simulink model "OffsetOutput_harness"  (Simulink 7.7)
settings: Solver=ode3  SolverMode=SingleTasking  StartTime=0.0  StopTime=25  FixedStep=.0005  RelTol=1e-3
PostLoadFcn:
  | cd '..';
  | PostLoadFcn;
  | cd 'harness';
InitFcn:
  | if signalbuilder('OffsetOutput_harness/Signal_Builder','activegroup') == 1
  |   CD_OFFSET_FUNCTION.DataType = 'uint8';
  |   CD_OFFSET_FUNCTION.Value = 255;
  | else
  |   CD_OFFSET_FUNCTION.DataType = 'uint8';
  |   CD_OFFSET_FUNCTION.Value = 0;
  | end
undefined symbols (not defined in the file): ACTIVE, BASE_ACTIVE, CD_PRECISION_REF_NOMINAL_VALUE, CD_VBATTERY_FILTER_DISPLAY_GAIN, CD_VBATTERY_FILTER_GAIN, CD_VBATTERY_GAIN, ENGINE_CRANKING, INIT_NORMAL, MXGTW_OFFSET, NON_FUNCTIONAL, ROD_ACTIVE, sigbuilder_block, srate, srate100, SYS_NORMAL
libraries: simulink x5, MX_Library x2
settings Model: Creator=smindema  LastModifiedBy=aliebel  CovPath=Offset  CovMetricSettings=dcmw  CovHTMLOptions=-aTS=1 -bRG=1 -bTC=1 -hTR=0 -nFC=0 -scm=1 -bcm=1 -xEv=0  covSaveCumulativeToWorkspaceVar=off  CovSaveSingleToWorkspaceVar=off
settings MATStruct: SampleTime=0.01  Offset=0  Priority=[1.0]
settings DataIOCC: LimitDataPoints=off  SaveOutput=off  SaveTime=off
settings OptimizationCC: BlockReduction=off  InlineParams=on  ExpressionFolding=off  StateBitsets=on  DataBitsets=on  UseTempVars=on  InitFltsAndDblsToZero=on  NoFixptDivByZeroProtection=on  EfficientFloat2IntCast=on  OptimizeModelRefInitCode=on
settings DebuggingCC: SaveWithParameterizedLinksMsg=none  MultiTaskDSMMsg=warning  MultiTaskCondExecSysMsg=none  IntegerOverflowMsg=none  ModelReferenceCSMismatchMessage=warning
settings HardwareCC: ProdBitPerInt=16  ProdBitPerPointer=16  ProdIntDivRoundTo=Floor  ProdEndianess=BigEndian  ProdWordSize=16  ProdHWDeviceType=Motorola HC12
settings ModelReferenceCC: ModelReferenceNumInstancesAllowed=Single
settings RTWCC: SystemTargetFile=ert.tlc  GenCodeOnly=on  TemplateMakefile=ert_default_tmf  Description=Real-Time Workshop Embedded Coder (no auto configuration)  GenerateReport=on  RetainRTWFile=on  ProcessScript=ert_make_rtw_hook  IncludeHyperlinkInReport=on  LaunchReport=on  IncludeERTFirstTime=on
settings RTWCC: CustomHeaderCode=|
  | #include "cpp_req_defines.h"
  | #include "hw_fin.h"
  | #include "cdata.h"
settings CodeAppCC: IgnoreCustomStorageClasses=off  DefineNamingRule=UpperCase
settings ERTTargetCC: TargetFcnLib=ansi_tfl_tmw.mat  FunctionExecutionProfile=off  MultiwordLength=2048  GenerateSampleERTMain=on  IncludeMdlTerminateFcn=off  SupportAbsoluteTime=off  SupportNonFinite=off  SupportComplex=off  PurelyIntegerCode=on  ERTCustomFileTemplate=gen_rtw_req_defines_h.tlc  GlobalDataDefinition=InSeparateSourceFile  GlobalDataReference=InSeparateHeaderFile  ConvertIfToSwitch=off

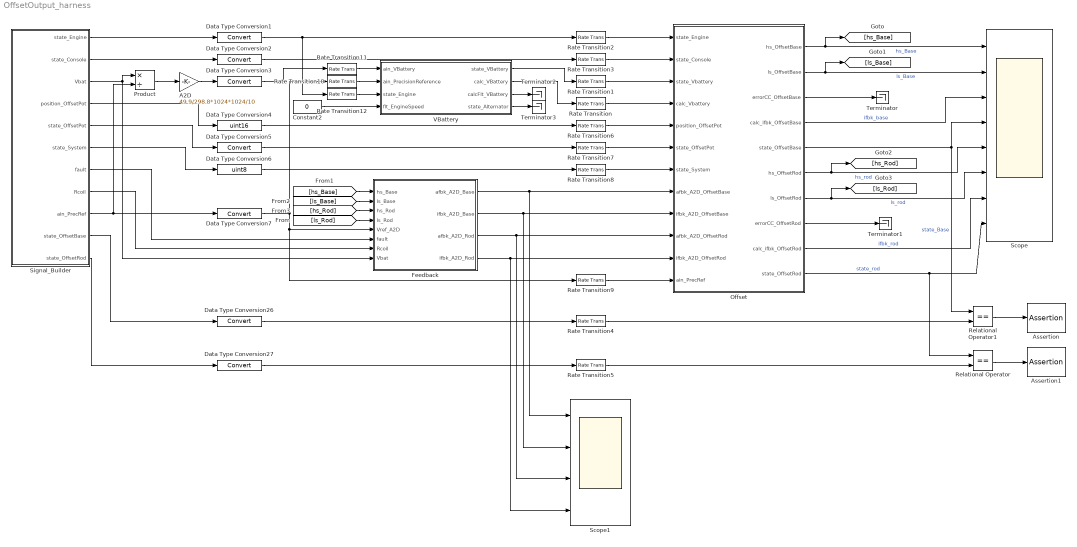
== system OffsetOutput_harness ==
  A2D : Gain  Gain=49.9/298.8*1024*1024/10  OutDataTypeStr=uint16
  Assertion : Assertion  Enabled=off
  Assertion1 : Assertion  Enabled=off
  Constant2 : Constant  Value=0  OutDataTypeStr=uint16
  Data Type Conversion{1..3,5,7,26..27} (7 alike) : DataTypeConversion
  Data Type Conversion4 : DataTypeConversion  OutDataTypeStr=uint16
  Data Type Conversion6 : DataTypeConversion  OutDataTypeStr=uint8
  Feedback : Subsystem
  Offset : Subsystem  TreatAsAtomicUnit=on  SystemSampleTime=srate  RTWFileName=mod_Outputs
      settings: RTWSystemCode=Function  RTWFcnNameOpts=Use subsystem name  RTWFileNameOpts=User specified
  Product : Product  Inputs=*/  RndMeth=Zero
  Rate Transition : RateTransition  X0=12
  Rate Transition1 : RateTransition  X0=8
  Rate Transition{2..12} (11 alike) : RateTransition
  Relational Operator : RelationalOperator  Operator===  OutDataTypeStr=boolean
  Relational Operator1 : RelationalOperator  Operator===  OutDataTypeStr=boolean
  Scope : Scope  NumInputPorts=8
      settings: TimeRange=50  YMin=0~0~0~0~0~0~0~0  YMax=0.3~1~1.25~1~0.4~1~1.5~1  DataFormat=Array
  Scope1 : Scope  NumInputPorts=4
      settings: TimeRange=100  YMin=0~0~0~0  YMax=6~10~6~60  SaveName=ScopeData2  DataFormat=Array
  Signal_Builder : Subsystem  Tag=STV Subsys  LoadFcn=sigbuilder_block('load');  StartFcn=sigbuilder_block('start');  StopFcn=sigbuilder_block('stop');  ClipboardFcn=sigbuilder_block('clipboard');  mask(Sigbuilder block){}
      mask help: Sigbuilder GUI
      mask init:
      | if ~strcmp(get_param(bdroot(gcbh),'SimulationStatus'),'stopped') tuvar = sigbuilder_block('maskInit'); end
      settings: CopyFcn=sigbuilder_block('copy');  DeleteFcn=sigbuilder_block('delete');  ModelCloseFcn=sigbuilder_block('modelClose');  PreSaveFcn=sigbuilder_block('preSave');  NameChangeFcn=sigbuilder_block('namechange');  OpenFcn=sigbuilder_block('open',[498.75 33 780.75 697.5 ]);  CloseFcn=sigbuilder_block('close');
      mask Display: plot(0,0,100,100,[10,10,40,40,10],[80,20,20,80,80],[40,10],[50,50], [40,27,10],[65,72,56],[40,25,25,10],[28,28,43,43]);
  Terminator{,1..3} (4 alike) : Terminator
  VBattery : Subsystem  TreatAsAtomicUnit=on  SystemSampleTime=srate100  RTWFileName=mod_Inputs
      settings: RTWSystemCode=Function  RTWFcnNameOpts=Use subsystem name  RTWFileNameOpts=User specified
  wires:
  Signal_Builder/2(state_Console) -> Data Type Conversion2/1
  Relational Operator/1 -> Assertion1/1
  Signal_Builder/1(state_Engine) -> Data Type Conversion1/1
  Signal_Builder/4(position_OffsetPot) -> Data Type Conversion4/1
  Relational Operator1/1 -> Assertion/1
  Signal_Builder/11(state_OffsetRod) -> Data Type Conversion27/1
  Data Type Conversion26/1 -> Rate Transition4/1
  Data Type Conversion27/1 -> Rate Transition5/1
  Data Type Conversion1/1 -> Rate Transition2/1, Rate Transition12/1
  Data Type Conversion2/1 -> Rate Transition3/1
  Signal_Builder/10(state_OffsetBase) -> Data Type Conversion26/1
  Data Type Conversion4/1 -> Rate Transition6/1
  Data Type Conversion5/1 -> Rate Transition7/1
  Data Type Conversion6/1 -> Rate Transition8/1
  Data Type Conversion7/1 -> Rate Transition10/1, Rate Transition9/1, Feedback/5(Vref_A2D)
  Signal_Builder/5(state_OffsetPot) -> Data Type Conversion5/1
  Signal_Builder/6(state_System) -> Data Type Conversion6/1
  Signal_Builder/9(ain_PrecRef) -> Data Type Conversion7/1, Product/2
  Offset/1(hs_OffsetBase) -> Scope/1, [hs_Base]  "hs_Base"
  Offset/2(ls_OffsetBase) -> Scope/2, [ls_Base]  "ls_Base"
  Offset/4(calc_ifbk_OffsetBase) -> Scope/3  "ifbk_base"
  Offset/5(state_OffsetBase) -> Scope/4, Relational Operator1/1  "state_Base"
  Offset/6(hs_OffsetRod) -> Scope/5, [hs_Rod]  "hs_rod"
  Offset/7(ls_OffsetRod) -> Scope/6, [ls_Rod]  "ls_rod"
  Offset/9(calc_ifbk_OffsetRod) -> Scope/7  "ifbk_rod"
  Offset/10(state_OffsetRod) -> Scope/8, Relational Operator/1  "state_rod"
  Offset/3(errorCC_OffsetBase) -> Terminator/1
  Offset/8(errorCC_OffsetRod) -> Terminator1/1
  VBattery/1(state_VBattery) -> Rate Transition1/1
  VBattery/2(calc_VBattery) -> Rate Transition/1
  VBattery/3(calcFlt_VBattery) -> Terminator2/1
  VBattery/4(state_Alternator) -> Terminator3/1
  Constant2/1 -> VBattery/4(flt_EngineSpeed)
  Signal_Builder/3(Vbat) -> Feedback/8(Vbat), Product/1
  A2D/1 -> Data Type Conversion3/1
  Data Type Conversion3/1 -> Rate Transition11/1
  Signal_Builder/7(fault) -> Feedback/6(fault)
  Signal_Builder/8(Rcoil) -> Feedback/7(Rcoil)
  [hs_Base] -> Feedback/1(hs_Base)
  [ls_Base] -> Feedback/2(ls_Base)
  [hs_Rod] -> Feedback/3(hs_Rod)
  [ls_Rod] -> Feedback/4(ls_Rod)
  Rate Transition1/1 -> Offset/3(state_Vbattery)
  Rate Transition/1 -> Offset/4(calc_Vbattery)
  Rate Transition2/1 -> Offset/1(state_Engine)
  Rate Transition3/1 -> Offset/2(state_Console)
  Rate Transition4/1 -> Relational Operator1/2
  Rate Transition5/1 -> Relational Operator/2
  Rate Transition6/1 -> Offset/5(position_OffsetPot)
  Rate Transition7/1 -> Offset/6(state_OffsetPot)
  Rate Transition8/1 -> Offset/7(state_System)
  Rate Transition9/1 -> Offset/12(ain_PrecRef)
  Rate Transition10/1 -> VBattery/2(ain_PrecisionReference)
  Rate Transition11/1 -> VBattery/1(ain_VBattery)
  Rate Transition12/1 -> VBattery/3(state_Engine)
  Feedback/1(afbk_A2D_Base) -> Offset/8(afbk_A2D_OffsetBase), Scope1/1
  Feedback/2(ifbk_A2D_Base) -> Offset/9(ifbk_A2D_OffsetBase), Scope1/2
  Feedback/3(afbk_A2D_Rod) -> Offset/10(afbk_A2D_OffsetRod), Scope1/3
  Feedback/4(ifbk_A2D_Rod) -> Offset/11(ifbk_A2D_OffsetRod), Scope1/4
  Product/1 -> A2D/1

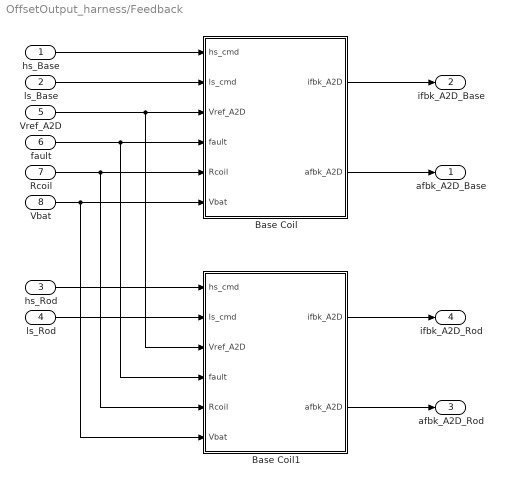
== system OffsetOutput_harness/Feedback ==
  hs_Base : Inport
  ls_Base : Inport  Port=2
  hs_Rod : Inport  Port=3
  ls_Rod : Inport  Port=4
  Vref_A2D : Inport  Port=5
  fault : Inport  Port=6
  Rcoil : Inport  Port=7
  Vbat : Inport  Port=8
  Base Coil : Subsystem
  Base Coil1 : Subsystem
  afbk_A2D_Base : Outport
  ifbk_A2D_Base : Outport  Port=2
  afbk_A2D_Rod : Outport  Port=3
  ifbk_A2D_Rod : Outport  Port=4
  wires:
  Base Coil/1(ifbk_A2D) -> ifbk_A2D_Base/1
  Base Coil/2(afbk_A2D) -> afbk_A2D_Base/1
  hs_Base/1 -> Base Coil/1(hs_cmd)
  ls_Base/1 -> Base Coil/2(ls_cmd)
  fault/1 -> Base Coil/4(fault), Base Coil1/4(fault)
  Rcoil/1 -> Base Coil/5(Rcoil), Base Coil1/5(Rcoil)
  Vbat/1 -> Base Coil/6(Vbat), Base Coil1/6(Vbat)
  Base Coil1/1(ifbk_A2D) -> ifbk_A2D_Rod/1
  Base Coil1/2(afbk_A2D) -> afbk_A2D_Rod/1
  hs_Rod/1 -> Base Coil1/1(hs_cmd)
  ls_Rod/1 -> Base Coil1/2(ls_cmd)
  Vref_A2D/1 -> Base Coil/3(Vref_A2D), Base Coil1/3(Vref_A2D)

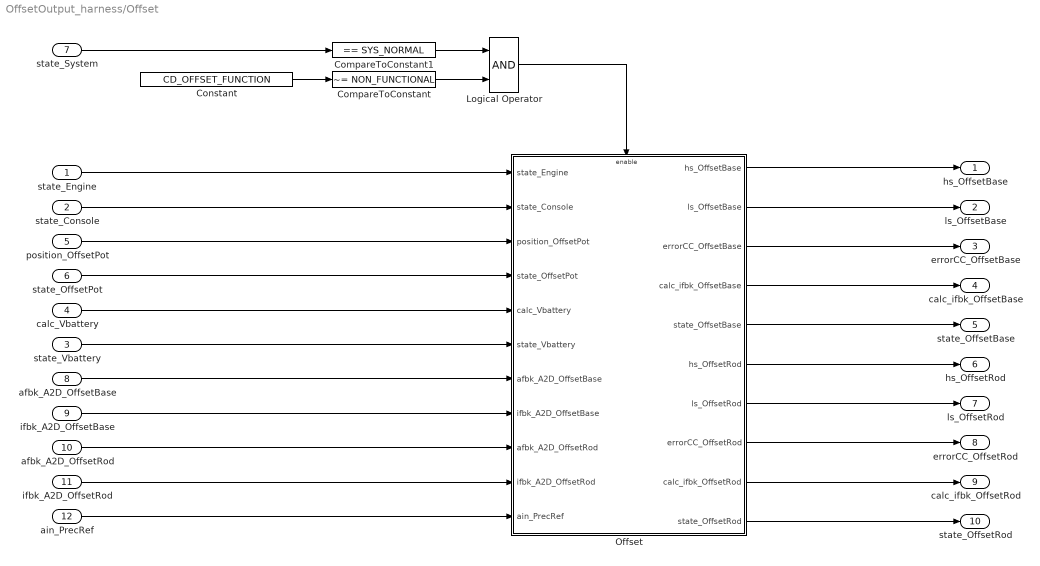
== system OffsetOutput_harness/Offset ==
  state_Engine : Inport
  state_Console : Inport  Port=2
  state_Vbattery : Inport  Port=3
  calc_Vbattery : Inport  Port=4
  position_OffsetPot : Inport  Port=5
  state_OffsetPot : Inport  Port=6
  state_System : Inport  Port=7
  afbk_A2D_OffsetBase : Inport  Port=8
  ifbk_A2D_OffsetBase : Inport  Port=9
  afbk_A2D_OffsetRod : Inport  Port=10
  ifbk_A2D_OffsetRod : Inport  Port=11
  ain_PrecRef : Inport  Port=12
  CompareToConstant : simulink/Logic and Bit Operations/Compare To Constant  SystemSampleTime=-1  relop=~=  const=NON_FUNCTIONAL  LogicOutDataTypeMode=boolean  ZeroCross=off
  CompareToConstant1 : simulink/Logic and Bit Operations/Compare To Constant  SystemSampleTime=-1  relop===  const=SYS_NORMAL  LogicOutDataTypeMode=boolean  ZeroCross=off
  Constant : Constant  Value=CD_OFFSET_FUNCTION
  Logical Operator : Logic  AllPortsSameDT=off  OutDataTypeStr=boolean
  Offset : Subsystem
  hs_OffsetBase : Outport  OutputWhenDisabled=reset  InitialOutput=[0]
  ls_OffsetBase : Outport  Port=2  OutputWhenDisabled=reset  InitialOutput=[0]
  errorCC_OffsetBase : Outport  Port=3  OutputWhenDisabled=reset  InitialOutput=[0]
  calc_ifbk_OffsetBase : Outport  Port=4  OutputWhenDisabled=reset  InitialOutput=[0]
  state_OffsetBase : Outport  Port=5  OutputWhenDisabled=reset  InitialOutput=[0]
  hs_OffsetRod : Outport  Port=6  OutputWhenDisabled=reset  InitialOutput=[0]
  ls_OffsetRod : Outport  Port=7  OutputWhenDisabled=reset  InitialOutput=[INIT_NORMAL]
  errorCC_OffsetRod : Outport  Port=8  OutputWhenDisabled=reset  InitialOutput=[0]
  calc_ifbk_OffsetRod : Outport  Port=9  OutputWhenDisabled=reset  InitialOutput=[INIT_NORMAL]
  state_OffsetRod : Outport  Port=10
  wires:
  state_System/1 -> CompareToConstant1/1
  CompareToConstant1/1 -> Logical Operator/1
  Constant/1 -> CompareToConstant/1
  CompareToConstant/1 -> Logical Operator/2
  Logical Operator/1 -> Offset/Enable
  state_Engine/1 -> Offset/1(state_Engine)
  state_Console/1 -> Offset/2(state_Console)
  position_OffsetPot/1 -> Offset/3(position_OffsetPot)
  state_OffsetPot/1 -> Offset/4(state_OffsetPot)
  calc_Vbattery/1 -> Offset/5(calc_Vbattery)
  state_Vbattery/1 -> Offset/6(state_Vbattery)
  afbk_A2D_OffsetBase/1 -> Offset/7(afbk_A2D_OffsetBase)
  ifbk_A2D_OffsetBase/1 -> Offset/8(ifbk_A2D_OffsetBase)
  afbk_A2D_OffsetRod/1 -> Offset/9(afbk_A2D_OffsetRod)
  ifbk_A2D_OffsetRod/1 -> Offset/10(ifbk_A2D_OffsetRod)
  Offset/1(hs_OffsetBase) -> hs_OffsetBase/1
  Offset/2(ls_OffsetBase) -> ls_OffsetBase/1
  Offset/3(errorCC_OffsetBase) -> errorCC_OffsetBase/1
  Offset/4(calc_ifbk_OffsetBase) -> calc_ifbk_OffsetBase/1
  Offset/5(state_OffsetBase) -> state_OffsetBase/1
  Offset/6(hs_OffsetRod) -> hs_OffsetRod/1
  Offset/7(ls_OffsetRod) -> ls_OffsetRod/1
  Offset/8(errorCC_OffsetRod) -> errorCC_OffsetRod/1
  Offset/9(calc_ifbk_OffsetRod) -> calc_ifbk_OffsetRod/1
  Offset/10(state_OffsetRod) -> state_OffsetRod/1
  ain_PrecRef/1 -> Offset/11(ain_PrecRef)

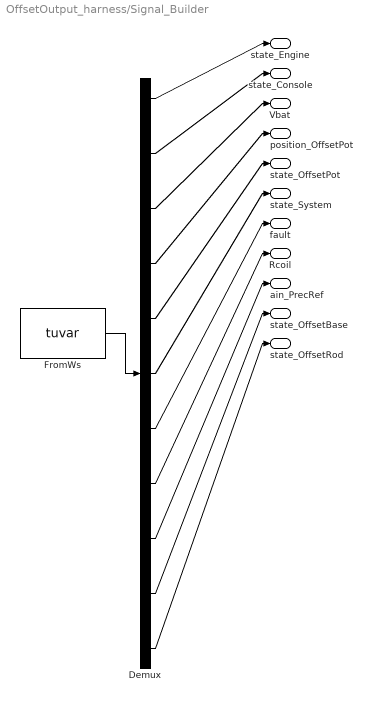
== system OffsetOutput_harness/Signal_Builder ==
  Demux : Demux  Tag=STV Demux  Outputs=11
  FromWs : FromWorkspace  Tag=STV FromWs  VariableName=tuvar  SampleTime=0  SigBuilderData=DataTag0  VnvData=DataTag1
      SigBuilderData=|
      | common.afterFinalStr = 'Extrapolate'
      | common.sampleTime = 0
      | dataSet(1).timeRange = [0 100]
      | dataSet(1).name = 'NonFunctional'
      | dataSet(2).timeRange = [0 100]
      | dataSet(2).name = 'Functional'
      | dataSet(3).timeRange = [0 100]
      | dataSet(3).name = 'Functional1'
      | dataSet(4).timeRange = [0 100]
      | dataSet(4).name = 'Open'
      | dataSet(5).timeRange = [0 100]
      | dataSet(5).name = 'STB'
      | dataSet(6).timeRange = [0 100]
      | dataSet(6).name = 'STG'
      | sbobj.Groups(1).Name = 'NonFunctional'
      | sbobj.Groups(1).Signals(1).Name = 'state_Engine'
      | sbobj.Groups(1).Signals(1).XData = [0 26 26 27 27 53 53 54 54 77 77 78 78 100]
      | sbobj.Groups(1).Signals(1).YData = [0 0 2 2 0 0 2 2 0 0 2 2 0 0]
      | sbobj.Groups(1).Signals(2).Name = 'state_Console'
      | sbobj.Groups(1).Signals(2).XData = [0 1 1 52 52 79 79 100]
      | sbobj.Groups(1).Signals(2).YData = [0 0 1 1 0 0 1 1]
      | sbobj.Groups(1).Signals(3).Name = 'Vbat'
      | sbobj.Groups(1).Signals(3).XData = [0 100]
      | sbobj.Groups(1).Signals(3).YData = [12 12]
      | sbobj.Groups(1).Signals(4).Name = 'position_OffsetPot'
      | sbobj.Groups(1).Signals(4).XData = [0 5 15 25 30 40 50 56 65 75 80 90 99 100]
      | sbobj.Groups(1).Signals(4).YData = [500 500 700 500 500 300 500 500 700 500 500 300 500 500]
      | sbobj.Groups(1).Signals(5).Name = 'state_OffsetPot'
      | sbobj.Groups(1).Signals(5).XData = [0 5 5 26 26 30 30 51 51 55 55 76 76 80 80 100]
      | sbobj.Groups(1).Signals(5).YData = [8 8 253 253 8 8 254 254 8 8 253 253 8 8 254 254]
      | sbobj.Groups(1).Signals(6).Name = 'state_System'
      | sbobj.Groups(1).Signals(6).XData = [0 78 78 100]
      | sbobj.Groups(1).Signals(6).YData = [1 1 2 2]
      | sbobj.Groups(1).Signals(7).Name = 'fault'
      | sbobj.Groups(1).Signals(7).XData = [0 100]
      | sbobj.Groups(1).Signals(7).YData = [0 0]
      | sbobj.Groups(1).Signals(8).Name = 'Rcoil'
      | sbobj.Groups(1).Signals(8).XData = [0 100]
      | sbobj.Groups(1).Signals(8).YData = [6 6]
      | sbobj.Groups(1).Signals(9).Name = 'ain_PrecRef'
      | sbobj.Groups(1).Signals(9).XData = [0 100]
      | sbobj.Groups(1).Signals(9).YData = [512 512]
      | sbobj.Groups(1).Signals(10).Name = 'state_OffsetBase'
      | sbobj.Groups(1).Signals(10).XData = [0 100]
      | sbobj.Groups(1).Signals(10).YData = [0 0]
      | sbobj.Groups(1).Signals(11).Name = 'state_OffsetRod'
      | sbobj.Groups(1).Signals(11).XData = [0 100]
      | sbobj.Groups(1).Signals(11).YData = [0 0]
      | sbobj.Groups(1).TimeRange = [0 100]
      | sbobj.Groups(2).Name = 'Functional'
      | sbobj.Groups(2).Signals(1).Name = 'state_Engine'
      | sbobj.Groups(2).Signals(1).XData = [0 26 26 27 27 53 53 54 54 77 77 78 78 100]
      | sbobj.Groups(2).Signals(1).YData = [0 0 2 2 0 0 2 2 0 0 2 2 0 0]
      | sbobj.Groups(2).Signals(2).Name = 'state_Console'
      | sbobj.Groups(2).Signals(2).XData = [0 1 1 52 52 79 79 100]
      | sbobj.Groups(2).Signals(2).YData = [0 0 1 1 0 0 1 1]
      | sbobj.Groups(2).Signals(3).Name = 'Vbat'
      | sbobj.Groups(2).Signals(3).XData = [0 100]
      | sbobj.Groups(2).Signals(3).YData = [12 12]
      | sbobj.Groups(2).Signals(4).Name = 'position_OffsetPot'
      | sbobj.Groups(2).Signals(4).XData = [0 5 15 25 30 40 50 56 65 75 80 90 99 100]
      | sbobj.Groups(2).Signals(4).YData = [500 500 700 500 500 300 500 500 700 500 500 300 500 500]
      | sbobj.Groups(2).Signals(5).Name = 'state_OffsetPot'
      | sbobj.Groups(2).Signals(5).XData = [0 5 5 26 26 30 30 51 51 55 55 76 76 80 80 100]
      | sbobj.Groups(2).Signals(5).YData = [8 8 253 253 8 8 254 254 8 8 253 253 8 8 254 254]
      | sbobj.Groups(2).Signals(6).Name = 'state_System'
      | sbobj.Groups(2).Signals(6).XData = [0 78 78 100]
      | sbobj.Groups(2).Signals(6).YData = [1 1 2 2]
      | sbobj.Groups(2).Signals(7).Name = 'fault'
      | sbobj.Groups(2).Signals(7).XData = [0 100]
      | sbobj.Groups(2).Signals(7).YData = [0 0]
      | sbobj.Groups(2).Signals(8).Name = 'Rcoil'
      | sbobj.Groups(2).Signals(8).XData = [0 100]
      | sbobj.Groups(2).Signals(8).YData = [6 6]
      | sbobj.Groups(2).Signals(9).Name = 'ain_PrecRef'
      | sbobj.Groups(2).Signals(9).XData = [0 100]
      | sbobj.Groups(2).Signals(9).YData = [512 512]
      | sbobj.Groups(2).Signals(10).Name = 'state_OffsetBase'
      | sbobj.Groups(2).Signals(10).XData = [0 6.85 6.85 23.16 23.16 100]
      | sbobj.Groups(2).Signals(10).YData = [0 0 1 1 0 0]
      | sbobj.Groups(2).Signals(11).Name = 'state_OffsetRod'
      | sbobj.Groups(2).Signals(11).XData = [0 77 77 88 88 100]
      | sbobj.Groups(2).Signals(11).YData = [0 0 1 1 0 0]
      | sbobj.Groups(2).TimeRange = [0 100]
      | sbobj.Groups(3).Name = 'Functional1'
      | sbobj.Groups(3).Signals(1).Name = 'state_Engine'
      | sbobj.Groups(3).Signals(1).XData = [0 70 70 90 90 100]
      | sbobj.Groups(3).Signals(1).YData = [0 0 2 2 1 1]
      | sbobj.Groups(3).Signals(2).Name = 'state_Console'
      | sbobj.Groups(3).Signals(2).XData = [0 1 1 22 22 26 26 100]
      | sbobj.Groups(3).Signals(2).YData = [0 0 1 1 0 0 1 1]
      | sbobj.Groups(3).Signals(3).Name = 'Vbat'
      | sbobj.Groups(3).Signals(3).XData = [0 74 74 94 94 100]
      | sbobj.Groups(3).Signals(3).YData = [12 12 5 5 14 14]
      | sbobj.Groups(3).Signals(4).Name = 'position_OffsetPot'
      | sbobj.Groups(3).Signals(4).XData = [0 3 3 5 5 7 7 9 9 34 34 57 57 100]
      | sbobj.Groups(3).Signals(4).YData = [500 500 600 600 400 400 600 600 500 500 400 400 500 500]
      | sbobj.Groups(3).Signals(5).Name = 'state_OffsetPot'
      | sbobj.Groups(3).Signals(5).XData = [0 3 3 5 5 7 7 9 9 18 18 58 58 76 80 100]
      | sbobj.Groups(3).Signals(5).YData = [8 8 253 253 254 254 253 253 8 8 254 254 8 8 8 8]
      | sbobj.Groups(3).Signals(6).Name = 'state_System'
      | sbobj.Groups(3).Signals(6).XData = [0 78 100]
      | sbobj.Groups(3).Signals(6).YData = [1 1 1]
      | sbobj.Groups(3).Signals(7).Name = 'fault'
      | sbobj.Groups(3).Signals(7).XData = [0 100]
      | sbobj.Groups(3).Signals(7).YData = [0 0]
      | sbobj.Groups(3).Signals(8).Name = 'Rcoil'
      | sbobj.Groups(3).Signals(8).XData = [0 100]
      | sbobj.Groups(3).Signals(8).YData = [6 6]
      | sbobj.Groups(3).Signals(9).Name = 'ain_PrecRef'
      | sbobj.Groups(3).Signals(9).XData = [0 34 34 44 44 56 56 100]
      | sbobj.Groups(3).Signals(9).YData = [512 512 400 400 600 600 512 512]
      | sbobj.Groups(3).Signals(10).Name = 'state_OffsetBase'
      | sbobj.Groups(3).Signals(10).XData = [0 100]
      | sbobj.Groups(3).Signals(10).YData = [0 0]
      | sbobj.Groups(3).Signals(11).Name = 'state_OffsetRod'
      | sbobj.Groups(3).Signals(11).XData = [0 100]
      | sbobj.Groups(3).Signals(11).YData = [0 0]
      | sbobj.Groups(3).TimeRange = [0 100]
      | sbobj.Groups(4).Name = 'Open'
      | sbobj.Groups(4).Signals(1).Name = 'state_Engine'
      | sbobj.Groups(4).Signals(1).XData = [0 70 90 100]
      | sbobj.Groups(4).Signals(1).YData = [0 0 0 0]
      | sbobj.Groups(4).Signals(2).Name = 'state_Console'
      | sbobj.Groups(4).Signals(2).XData = [0 10 10 22 56 56 62 62 100]
      | sbobj.Groups(4).Signals(2).YData = [0 0 1 1 1 0 0 1 1]
      | sbobj.Groups(4).Signals(3).Name = 'Vbat'
      | sbobj.Groups(4).Signals(3).XData = [0 74 94 100]
      | sbobj.Groups(4).Signals(3).YData = [12 12 12 12]
      | sbobj.Groups(4).Signals(4).Name = 'position_OffsetPot'
      | sbobj.Groups(4).Signals(4).XData = [0 15 15 23 23 30 30 37 37 64 64 84 84 100]
      | sbobj.Groups(4).Signals(4).YData = [500 500 600 600 500 500 400 400 500 500 600 600 500 500]
      | sbobj.Groups(4).Signals(5).Name = 'state_OffsetPot'
      | sbobj.Groups(4).Signals(5).XData = [0 15 15 23 23 30 30 37 37 64 64 84 84 100]
      | sbobj.Groups(4).Signals(5).YData = [8 8 253 253 8 8 254 254 8 8 253 253 8 8]
      | sbobj.Groups(4).Signals(6).Name = 'state_System'
      | sbobj.Groups(4).Signals(6).XData = [0 8 8 9 9 12 12 13 13 24 24 25 25 39 39 40 40 78 100]
      | sbobj.Groups(4).Signals(6).YData = [1 1 0 0 1 1 0 0 1 1 0 0 1 1 0 0 1 1 1]
      | sbobj.Groups(4).Signals(7).Name = 'fault'
      | sbobj.Groups(4).Signals(7).XData = [0 5 5 8 8 10 10 12 12 14 14 14.05 14.05 17.91 17.91 20.09 20.09 31.64 31.64 34.2 34.2 100]
      | sbobj.Groups(4).Signals(7).YData = [0 0 1 1 0 0 1 1 0 0 1 1 0 0 1 1 0 0 1 1 0 0]
      | sbobj.Groups(4).Signals(8).Name = 'Rcoil'
      | sbobj.Groups(4).Signals(8).XData = [0 51.8 51.8 100]
      | sbobj.Groups(4).Signals(8).YData = [6 6 200 200]
      | sbobj.Groups(4).Signals(9).Name = 'ain_PrecRef'
      | sbobj.Groups(4).Signals(9).XData = [0 100]
      | sbobj.Groups(4).Signals(9).YData = [512 512]
      | sbobj.Groups(4).Signals(10).Name = 'state_OffsetBase'
      | sbobj.Groups(4).Signals(10).XData = [0 100]
      | sbobj.Groups(4).Signals(10).YData = [0 0]
      | sbobj.Groups(4).Signals(11).Name = 'state_OffsetRod'
      | sbobj.Groups(4).Signals(11).XData = [0 100]
      | sbobj.Groups(4).Signals(11).YData = [0 0]
      | sbobj.Groups(4).TimeRange = [0 100]
      | sbobj.Groups(5).Name = 'STB'
      | sbobj.Groups(5).Signals(1).Name = 'state_Engine'
      | sbobj.Groups(5).Signals(1).XData = [0 70 90 100]
      | sbobj.Groups(5).Signals(1).YData = [0 0 0 0]
      | sbobj.Groups(5).Signals(2).Name = 'state_Console'
      | sbobj.Groups(5).Signals(2).XData = [0 10 10 22 26 40 40 43 43 100]
      | sbobj.Groups(5).Signals(2).YData = [0 0 1 1 1 1 0 0 1 1]
      | sbobj.Groups(5).Signals(3).Name = 'Vbat'
      | sbobj.Groups(5).Signals(3).XData = [0 74 94 100]
      | sbobj.Groups(5).Signals(3).YData = [12 12 12 12]
      | sbobj.Groups(5).Signals(4).Name = 'position_OffsetPot'
      | sbobj.Groups(5).Signals(4).XData = [0 15 15 23 23 30 30 37 37 52 52 59 59 62 62 68 68 100]
      | sbobj.Groups(5).Signals(4).YData = [500 500 600 600 500 500 400 400 500 500 600 600 500 500 400 400 500 500]
      | sbobj.Groups(5).Signals(5).Name = 'state_OffsetPot'
      | sbobj.Groups(5).Signals(5).XData = [0 15 15 23 23 30 30 37 37 52 52 59 59 62 62 68 68 100]
      | sbobj.Groups(5).Signals(5).YData = [8 8 253 253 8 8 254 254 8 8 253 253 8 8 254 254 8 8]
      | sbobj.Groups(5).Signals(6).Name = 'state_System'
      | sbobj.Groups(5).Signals(6).XData = [0 8 8 9 9 12 12 13 13 24 24 25 25 39 39 40 40 43 43 44 44 47 47 48 48 58 58 59 59 67 67 68 68 100]
      | sbobj.Groups(5).Signals(6).YData = [1 1 0 0 1 1 0 0 1 1 0 0 1 1 0 0 1 1 0 0 1 1 0 0 1 1 0 0 1 1 0 0 1 1]
      | sbobj.Groups(5).Signals(7).Name = 'fault'
      | sbobj.Groups(5).Signals(7).XData = [0 5 5 8 8 10 10 12 12 14 14 14.01 14.01 17.91 17.91 20.09 20.09 31.64 31.64 34.2 34.2 41.39 41.39 43.05 43.05 44.85 44.85 46.77 46.77 50 50 50.01 50.01 54.21 54.21 56.9 56.9 63.96 63.96 66.4 66.4 100]
      | sbobj.Groups(5).Signals(7).YData = [0 0 2 2 0 0 2 2 0 0 2 2 0 0 2 2 0 0 2 2 0 0 3 3 0 0 3 3 0 0 3 3 0 0 3 3 0 0 3 3 0 0]
      | sbobj.Groups(5).Signals(8).Name = 'Rcoil'
      | sbobj.Groups(5).Signals(8).XData = [0 100]
      | sbobj.Groups(5).Signals(8).YData = [6 6]
      | sbobj.Groups(5).Signals(9).Name = 'ain_PrecRef'
      | sbobj.Groups(5).Signals(9).XData = [0 100]
      | sbobj.Groups(5).Signals(9).YData = [512 512]
      | sbobj.Groups(5).Signals(10).Name = 'state_OffsetBase'
      | sbobj.Groups(5).Signals(10).XData = [0 100]
      | sbobj.Groups(5).Signals(10).YData = [0 0]
      | sbobj.Groups(5).Signals(11).Name = 'state_OffsetRod'
      | sbobj.Groups(5).Signals(11).XData = [0 100]
      | sbobj.Groups(5).Signals(11).YData = [0 0]
      | sbobj.Groups(5).TimeRange = [0 100]
      | sbobj.Groups(6).Name = 'STG'
      | sbobj.Groups(6).Signals(1).Name = 'state_Engine'
      | sbobj.Groups(6).Signals(1).XData = [0 70 90 100]
      | sbobj.Groups(6).Signals(1).YData = [0 0 0 0]
      | sbobj.Groups(6).Signals(2).Name = 'state_Console'
      | sbobj.Groups(6).Signals(2).XData = [0 10 10 22 26 40 40 43 43 100]
      | sbobj.Groups(6).Signals(2).YData = [0 0 1 1 1 1 0 0 1 1]
      | sbobj.Groups(6).Signals(3).Name = 'Vbat'
      | sbobj.Groups(6).Signals(3).XData = [0 74 94 100]
      | sbobj.Groups(6).Signals(3).YData = [12 12 12 12]
      | sbobj.Groups(6).Signals(4).Name = 'position_OffsetPot'
      | sbobj.Groups(6).Signals(4).XData = [0 15 15 23 23 30 30 37 37 52 52 59 59 62 62 68 68 100]
      | sbobj.Groups(6).Signals(4).YData = [500 500 600 600 500 500 400 400 500 500 600 600 500 500 400 400 500 500]
      | sbobj.Groups(6).Signals(5).Name = 'state_OffsetPot'
      | sbobj.Groups(6).Signals(5).XData = [0 15 15 23 23 30 30 37 37 52 52 59 59 62 62 68 68 100]
      | sbobj.Groups(6).Signals(5).YData = [8 8 253 253 8 8 254 254 8 8 253 253 8 8 254 254 8 8]
      | sbobj.Groups(6).Signals(6).Name = 'state_System'
      | sbobj.Groups(6).Signals(6).XData = [0 8 8 9 9 12 12 13 13 24 24 25 25 39 39 40 40 43 43 44 44 47 47 48 48 58 58 59 59 67 67 68 68 100]
      | sbobj.Groups(6).Signals(6).YData = [1 1 0 0 1 1 0 0 1 1 0 0 1 1 0 0 1 1 0 0 1 1 0 0 1 1 0 0 1 1 0 0 1 1]
      | sbobj.Groups(6).Signals(7).Name = 'fault'
      | sbobj.Groups(6).Signals(7).XData = [0 5 5 8 8 10 10 12 12 14 14 14.01 14.01 17.91 17.91 20.09 20.09 31.64 31.64 34.2 34.2 41.39 41.39 43.05 43.05 44.85 44.85 46.77 46.77 50 50 50.01 50.01 54.21 54.21 56.9 56.9 63.96 63.96 66.4 66.4 100]
      | sbobj.Groups(6).Signals(7).YData = [0 0 4 4 0 0 4 4 0 0 4 4 0 0 4 4 0 0 4 4 0 0 5 5 0 0 5 5 0 0 5 5 0 0 5 5 0 0 5 5 0 0]
      | sbobj.Groups(6).Signals(8).Name = 'Rcoil'
      | sbobj.Groups(6).Signals(8).XData = [0 100]
      | sbobj.Groups(6).Signals(8).YData = [6 6]
      | sbobj.Groups(6).Signals(9).Name = 'ain_PrecRef'
      | sbobj.Groups(6).Signals(9).XData = [0 100]
      | sbobj.Groups(6).Signals(9).YData = [512 512]
      | sbobj.Groups(6).Signals(10).Name = 'state_OffsetBase'
      | sbobj.Groups(6).Signals(10).XData = [0 100]
      | sbobj.Groups(6).Signals(10).YData = [0 0]
      | sbobj.Groups(6).Signals(11).Name = 'state_OffsetRod'
      | sbobj.Groups(6).Signals(11).XData = [0 100]
      | sbobj.Groups(6).Signals(11).YData = [0 0]
      | sbobj.Groups(6).TimeRange = [0 100]
  state_Engine : Outport  Tag=STV Outport
  state_Console : Outport  Tag=STV Outport  Port=2
  Vbat : Outport  Tag=STV Outport  Port=3
  position_OffsetPot : Outport  Tag=STV Outport  Port=4
  state_OffsetPot : Outport  Tag=STV Outport  Port=5
  state_System : Outport  Tag=STV Outport  Port=6
  fault : Outport  Tag=STV Outport  Port=7
  Rcoil : Outport  Tag=STV Outport  Port=8
  ain_PrecRef : Outport  Tag=STV Outport  Port=9
  state_OffsetBase : Outport  Tag=STV Outport  Port=10
  state_OffsetRod : Outport  Tag=STV Outport  Port=11
  wires:
  FromWs/1 -> Demux/1
  Demux/1 -> state_Engine/1
  Demux/2 -> state_Console/1
  Demux/3 -> Vbat/1
  Demux/4 -> position_OffsetPot/1
  Demux/5 -> state_OffsetPot/1
  Demux/6 -> state_System/1
  Demux/7 -> fault/1
  Demux/8 -> Rcoil/1
  Demux/9 -> ain_PrecRef/1
  Demux/10 -> state_OffsetBase/1
  Demux/11 -> state_OffsetRod/1

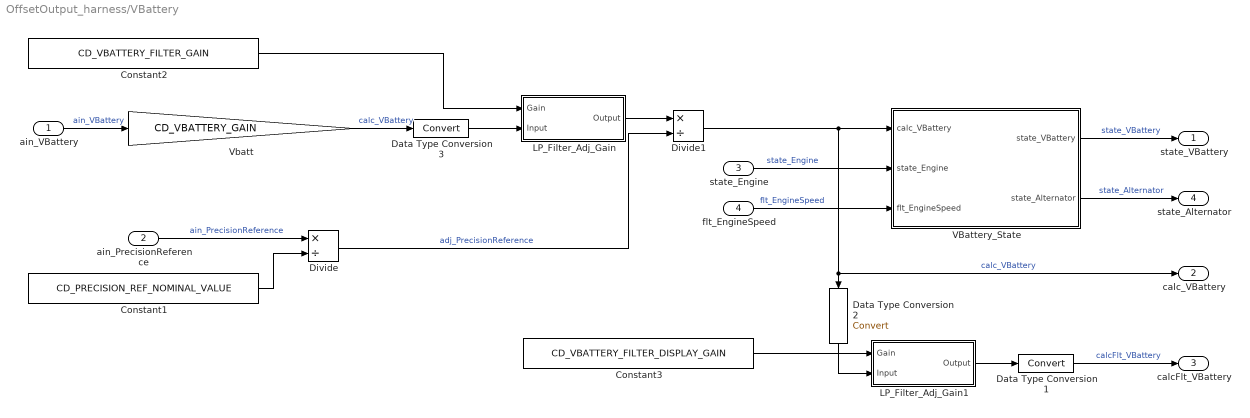
== system OffsetOutput_harness/VBattery ==
  ain_VBattery : Inport  OutDataTypeStr=uint16
  ain_PrecisionReference : Inport  Port=2  OutDataTypeStr=uint16
  state_Engine : Inport  Port=3
  flt_EngineSpeed : Inport  Port=4  OutDataTypeStr=uint16
  Constant1 : Constant  Value=CD_PRECISION_REF_NOMINAL_VALUE  OutDataTypeStr=uint16  SampleTime=srate100
  Constant2 : Constant  Value=CD_VBATTERY_FILTER_GAIN  OutDataTypeStr=uint8  SampleTime=srate100
  Constant3 : Constant  Value=CD_VBATTERY_FILTER_DISPLAY_GAIN  OutDataTypeStr=uint8  SampleTime=srate100
  Data Type Conversion1 : DataTypeConversion
  Data Type Conversion2 : DataTypeConversion
  Data Type Conversion3 : DataTypeConversion
  Divide : Product  Inputs=*/  OutDataTypeStr=fixdt(0,16,10)  RndMeth=Nearest
  Divide1 : Product  Inputs=*/  OutDataTypeStr=fixdt(0,16,8)  RndMeth=Nearest
  LP_Filter_Adj_Gain : Subsystem
  LP_Filter_Adj_Gain1 : Subsystem
  VBattery_State : Stateflow chart  TreatAsAtomicUnit=on
  Vbatt : Gain  Gain=CD_VBATTERY_GAIN  ParamDataTypeStr=fixdt(0,16,12)  OutDataTypeStr=fixdt(0,16,8)  RndMeth=Nearest  SampleTime=srate100  SaturateOnIntegerOverflow=on
  state_VBattery : Outport  OutDataTypeStr=uint8
  calc_VBattery : Outport  Port=2
  calcFlt_VBattery : Outport  Port=3  OutDataTypeStr=fixdt(0,16,8)
  state_Alternator : Outport  Port=4  OutDataTypeStr=uint8
  wires:
  ain_VBattery/1 -> Vbatt/1  "ain_VBattery"
  state_Engine/1 -> VBattery_State/2(state_Engine)  "state_Engine"
  Data Type Conversion1/1 -> calcFlt_VBattery/1  "calcFlt_VBattery"
  LP_Filter_Adj_Gain1/1(Output) -> Data Type Conversion1/1
  ain_PrecisionReference/1 -> Divide/1  "ain_PrecisionReference"
  Constant1/1 -> Divide/2
  Divide/1 -> Divide1/2  "adj_PrecisionReference"
  Vbatt/1 -> Data Type Conversion3/1  "calc_VBattery"
  Divide1/1 -> VBattery_State/1(calc_VBattery), calc_VBattery/1, Data Type Conversion2/1  "calc_VBattery"
  LP_Filter_Adj_Gain/1(Output) -> Divide1/1
  flt_EngineSpeed/1 -> VBattery_State/3(flt_EngineSpeed)  "flt_EngineSpeed"
  VBattery_State/1(state_VBattery) -> state_VBattery/1  "state_VBattery"
  VBattery_State/2(state_Alternator) -> state_Alternator/1  "state_Alternator"
  Constant2/1 -> LP_Filter_Adj_Gain/1(Gain)
  Constant3/1 -> LP_Filter_Adj_Gain1/1(Gain)
  Data Type Conversion2/1 -> LP_Filter_Adj_Gain1/2(Input)
  Data Type Conversion3/1 -> LP_Filter_Adj_Gain/2(Input)

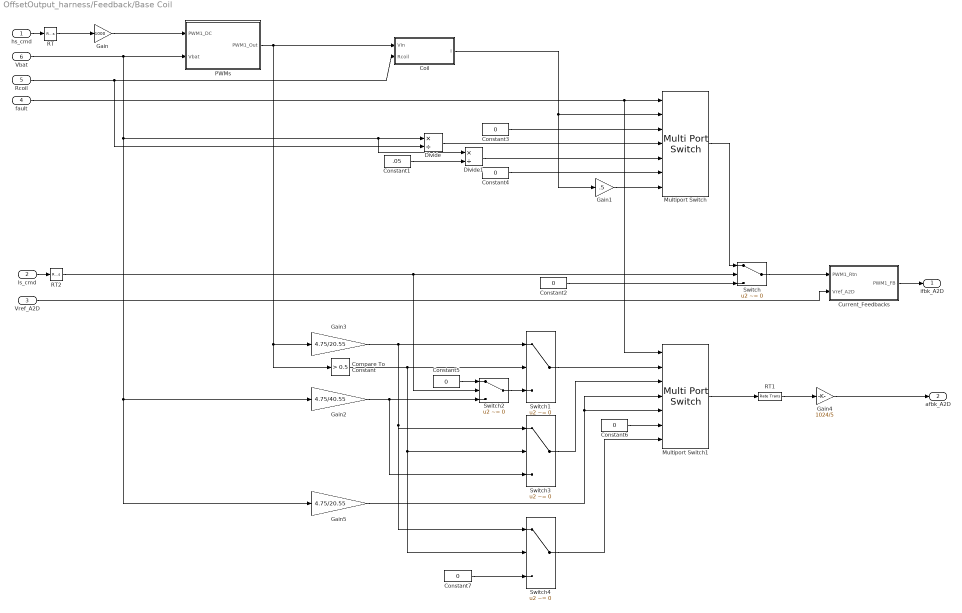
== system OffsetOutput_harness/Feedback/Base Coil ==
  hs_cmd : Inport
  ls_cmd : Inport  Port=2
  Vref_A2D : Inport  Port=3
  fault : Inport  Port=4
  Rcoil : Inport  Port=5
  Vbat : Inport  Port=6
  Coil : Subsystem
  Compare To Constant : simulink/Logic and Bit Operations/Compare To Constant  SystemSampleTime=-1  relop=>  const=0.5  LogicOutDataTypeMode=boolean
  Constant1 : Constant  Value=.05
  Constant{2..7} (6 alike) : Constant  Value=0
  Current_Feedbacks : Subsystem
  Divide : Product  Inputs=*/
  Divide1 : Product  Inputs=*/
  Gain : Gain  Gain=1000
  Gain1 : Gain  Gain=.5
  Gain2 : Gain  Gain=4.75/40.55
  Gain3 : Gain  Gain=4.75/20.55
  Gain4 : Gain  Gain=1024/5  OutDataTypeStr=uint16
  Gain5 : Gain  Gain=4.75/20.55
  Multiport Switch : MultiPortSwitch  DataPortOrder=Zero-based contiguous  Inputs=6  zeroidx=on
  Multiport Switch1 : MultiPortSwitch  DataPortOrder=Zero-based contiguous  Inputs=6  zeroidx=on
  PWMs : Subsystem
  RT : RateTransition  OutPortSampleTime=0
  RT1 : RateTransition  OutPortSampleTime=.01
  RT2 : RateTransition  OutPortSampleTime=0
  Switch{,1..4} (5 alike) : Switch  Criteria=u2 ~= 0
  ifbk_A2D : Outport
  afbk_A2D : Outport  Port=2
  wires:
  Vbat/1 -> PWMs/2(Vbat), Divide/1, Divide1/1, Gain5/1, Gain2/1
  PWMs/1(PWM1_Out) -> Coil/1(Vin), Gain3/1, Compare To Constant/1
  Gain/1 -> PWMs/1(PWM1_DC)
  hs_cmd/1 -> RT/1
  RT/1 -> Gain/1
  ls_cmd/1 -> RT2/1
  Constant2/1 -> Switch/3
  fault/1 -> Multiport Switch/1, Multiport Switch1/1
  Constant3/1 -> Multiport Switch/3
  Multiport Switch/1 -> Switch/1
  Rcoil/1 -> Coil/2(Rcoil), Divide/2
  Current_Feedbacks/1(PWM1_FB) -> ifbk_A2D/1
  Switch/1 -> Current_Feedbacks/1(PWM1_Rtn)
  Coil/1(I) -> Multiport Switch/2, Gain1/1
  Divide/1 -> Multiport Switch/4
  Divide1/1 -> Multiport Switch/5
  Constant1/1 -> Divide1/2
  Constant4/1 -> Multiport Switch/6
  Gain1/1 -> Multiport Switch/7
  Compare To Constant/1 -> Switch1/2, Switch3/2, Switch4/2
  Gain3/1 -> Switch1/1, Switch3/1, Switch4/1
  Switch1/1 -> Multiport Switch1/2
  Switch2/1 -> Switch1/3
  Constant5/1 -> Switch2/1
  Gain2/1 -> Switch2/3, Switch3/3
  Multiport Switch1/1 -> RT1/1
  Gain4/1 -> afbk_A2D/1
  Switch3/1 -> Multiport Switch1/3
  Gain5/1 -> Multiport Switch1/4, Multiport Switch1/5
  Constant6/1 -> Multiport Switch1/6
  Constant7/1 -> Switch4/3
  Switch4/1 -> Multiport Switch1/7
  RT1/1 -> Gain4/1
  RT2/1 -> Switch/2, Switch2/2
  Vref_A2D/1 -> Current_Feedbacks/2(Vref_A2D)

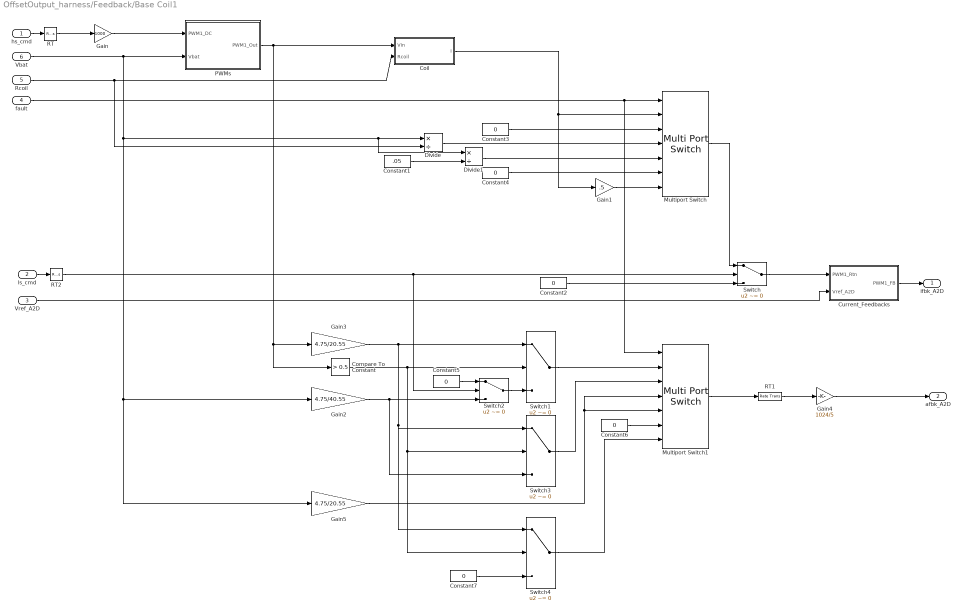
== system OffsetOutput_harness/Feedback/Base Coil1 ==
  hs_cmd : Inport
  ls_cmd : Inport  Port=2
  Vref_A2D : Inport  Port=3
  fault : Inport  Port=4
  Rcoil : Inport  Port=5
  Vbat : Inport  Port=6
  Coil : Subsystem
  Compare To Constant : simulink/Logic and Bit Operations/Compare To Constant  SystemSampleTime=-1  relop=>  const=0.5  LogicOutDataTypeMode=boolean
  Constant1 : Constant  Value=.05
  Constant{2..7} (6 alike) : Constant  Value=0
  Current_Feedbacks : Subsystem
  Divide : Product  Inputs=*/
  Divide1 : Product  Inputs=*/
  Gain : Gain  Gain=1000
  Gain1 : Gain  Gain=.5
  Gain2 : Gain  Gain=4.75/40.55
  Gain3 : Gain  Gain=4.75/20.55
  Gain4 : Gain  Gain=1024/5  OutDataTypeStr=uint16
  Gain5 : Gain  Gain=4.75/20.55
  Multiport Switch : MultiPortSwitch  DataPortOrder=Zero-based contiguous  Inputs=6  zeroidx=on
  Multiport Switch1 : MultiPortSwitch  DataPortOrder=Zero-based contiguous  Inputs=6  zeroidx=on
  PWMs : Subsystem
  RT : RateTransition  OutPortSampleTime=0
  RT1 : RateTransition  OutPortSampleTime=.01
  RT2 : RateTransition  OutPortSampleTime=0
  Switch{,1..4} (5 alike) : Switch  Criteria=u2 ~= 0
  ifbk_A2D : Outport
  afbk_A2D : Outport  Port=2
  wires:
  Vbat/1 -> PWMs/2(Vbat), Divide/1, Divide1/1, Gain5/1, Gain2/1
  PWMs/1(PWM1_Out) -> Coil/1(Vin), Gain3/1, Compare To Constant/1
  Gain/1 -> PWMs/1(PWM1_DC)
  hs_cmd/1 -> RT/1
  RT/1 -> Gain/1
  ls_cmd/1 -> RT2/1
  Constant2/1 -> Switch/3
  fault/1 -> Multiport Switch/1, Multiport Switch1/1
  Constant3/1 -> Multiport Switch/3
  Multiport Switch/1 -> Switch/1
  Rcoil/1 -> Coil/2(Rcoil), Divide/2
  Current_Feedbacks/1(PWM1_FB) -> ifbk_A2D/1
  Switch/1 -> Current_Feedbacks/1(PWM1_Rtn)
  Coil/1(I) -> Multiport Switch/2, Gain1/1
  Divide/1 -> Multiport Switch/4
  Divide1/1 -> Multiport Switch/5
  Constant1/1 -> Divide1/2
  Constant4/1 -> Multiport Switch/6
  Gain1/1 -> Multiport Switch/7
  Compare To Constant/1 -> Switch1/2, Switch3/2, Switch4/2
  Gain3/1 -> Switch1/1, Switch3/1, Switch4/1
  Switch1/1 -> Multiport Switch1/2
  Switch2/1 -> Switch1/3
  Constant5/1 -> Switch2/1
  Gain2/1 -> Switch2/3, Switch3/3
  Multiport Switch1/1 -> RT1/1
  Gain4/1 -> afbk_A2D/1
  Switch3/1 -> Multiport Switch1/3
  Gain5/1 -> Multiport Switch1/4, Multiport Switch1/5
  Constant6/1 -> Multiport Switch1/6
  Constant7/1 -> Switch4/3
  Switch4/1 -> Multiport Switch1/7
  RT1/1 -> Gain4/1
  RT2/1 -> Switch/2, Switch2/2
  Vref_A2D/1 -> Current_Feedbacks/2(Vref_A2D)

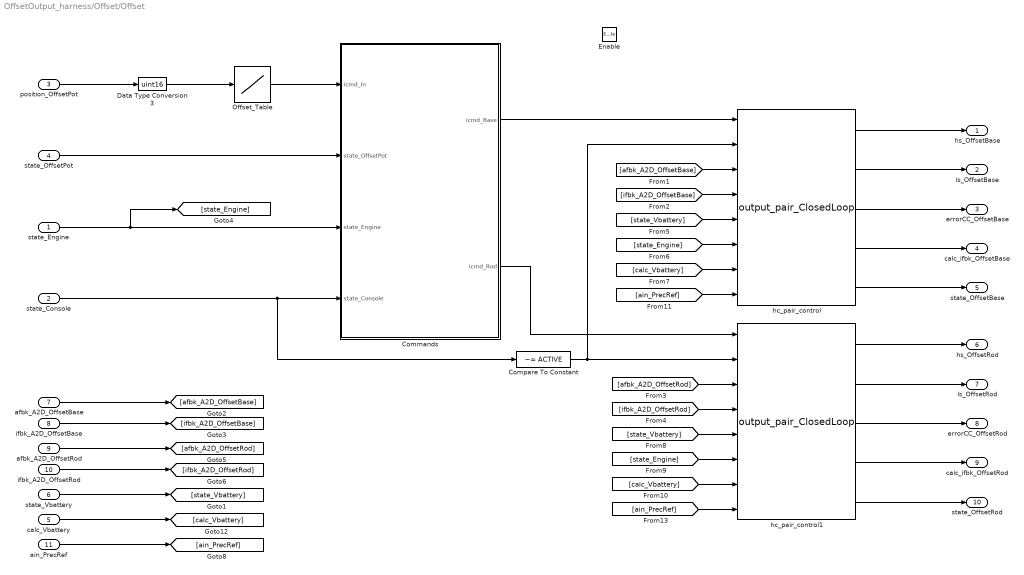
== system OffsetOutput_harness/Offset/Offset ==
  state_Engine : Inport
  state_Console : Inport  Port=2
  position_OffsetPot : Inport  Port=3
  state_OffsetPot : Inport  Port=4
  calc_Vbattery : Inport  Port=5
  state_Vbattery : Inport  Port=6
  afbk_A2D_OffsetBase : Inport  Port=7
  ifbk_A2D_OffsetBase : Inport  Port=8
  afbk_A2D_OffsetRod : Inport  Port=9
  ifbk_A2D_OffsetRod : Inport  Port=10
  ain_PrecRef : Inport  Port=11
  Enable : EnablePort  StatesWhenEnabling=reset  PropagateVarSize=During execution
  Commands : Stateflow chart  TreatAsAtomicUnit=on
  Compare To Constant : simulink/Logic and Bit Operations/Compare To Constant  SystemSampleTime=-1  relop=~=  const=ACTIVE  LogicOutDataTypeMode=boolean
  Data Type Conversion3 : DataTypeConversion  OutDataTypeStr=uint16
  Offset_Table : Lookup  InputValues=[20:6:980]  Table=MXGTW_OFFSET  LookUpMeth=Interpolation-Use End Values  OutDataTypeStr=fixdt(0,16,12)  SaturateOnIntegerOverflow=on
      settings: AttributesFormatString=input = %<InputValues>\noutput = %<OutputValues>
  hc_pair_control : MX_Library/output_pair_ClosedLoop  SystemSampleTime=-1  AFBK_GAIN=CD_OFFSET_AFBK_GAIN  IFBK_GAIN=CD_OFFSET_IFBK_GAIN  OPEN_DB_CNT=CD_OFFSET_DEBOUNCE_OPEN_CIRCUIT  STG_DB_CNT=CD_OFFSET_DEBOUNCE_SHORT_TO_GROUND  OSTG_DB_CNT=CD_OFFSET_DEBOUNCE_SHORT_TO_GROUND  STB_DB_CNT=CD_OFFSET_DEBOUNCE_SHORT_TO_BATTERY  OC_DB_CNT=CD_OFFSET_DEBOUNCE_OVERCURRENT  IFBK_MAX=CD_OFFSET_OVERCURRENT  NZ_IFBK=CD_OFFSET_NON_ZERO_CURRENT  NZ_DUTY=CD_OFFSET_NON_ZERO_DUTY  KP=CD_OFFSET_KP  KI=CD_OFFSET_KI
  hc_pair_control1 : MX_Library/output_pair_ClosedLoop  SystemSampleTime=-1  AFBK_GAIN=CD_OFFSET_AFBK_GAIN  IFBK_GAIN=CD_OFFSET_IFBK_GAIN  OPEN_DB_CNT=CD_OFFSET_DEBOUNCE_OPEN_CIRCUIT  STG_DB_CNT=CD_OFFSET_DEBOUNCE_SHORT_TO_GROUND  OSTG_DB_CNT=CD_OFFSET_DEBOUNCE_SHORT_TO_GROUND  STB_DB_CNT=CD_OFFSET_DEBOUNCE_SHORT_TO_BATTERY  OC_DB_CNT=CD_OFFSET_DEBOUNCE_OVERCURRENT  IFBK_MAX=CD_OFFSET_OVERCURRENT  NZ_IFBK=CD_OFFSET_NON_ZERO_CURRENT  NZ_DUTY=CD_OFFSET_NON_ZERO_DUTY  KP=CD_OFFSET_KP  KI=CD_OFFSET_KI
  hs_OffsetBase : Outport  OutputWhenDisabled=reset  InitialOutput=[0]
  ls_OffsetBase : Outport  Port=2  OutputWhenDisabled=reset  InitialOutput=[0]
  errorCC_OffsetBase : Outport  Port=3  OutputWhenDisabled=reset  InitialOutput=[0]
  calc_ifbk_OffsetBase : Outport  Port=4  OutputWhenDisabled=reset  InitialOutput=[0]
  state_OffsetBase : Outport  Port=5  OutputWhenDisabled=reset  InitialOutput=[0]
  hs_OffsetRod : Outport  Port=6  OutputWhenDisabled=reset  InitialOutput=[0]
  ls_OffsetRod : Outport  Port=7  OutputWhenDisabled=reset  InitialOutput=[0]
  errorCC_OffsetRod : Outport  Port=8  OutputWhenDisabled=reset  InitialOutput=[0]
  calc_ifbk_OffsetRod : Outport  Port=9  OutputWhenDisabled=reset  InitialOutput=[0]
  state_OffsetRod : Outport  Port=10  InitialOutput=[0]
  wires:
  position_OffsetPot/1 -> Data Type Conversion3/1
  state_Engine/1 -> Commands/3(state_Engine), [state_Engine]
  state_OffsetPot/1 -> Commands/2(state_OffsetPot)
  Offset_Table/1 -> Commands/1(icmd_In)
  state_Console/1 -> Commands/4(state_Console), Compare To Constant/1
  Data Type Conversion3/1 -> Offset_Table/1
  afbk_A2D_OffsetBase/1 -> [afbk_A2D_OffsetBase]
  ifbk_A2D_OffsetBase/1 -> [ifbk_A2D_OffsetBase]
  state_Vbattery/1 -> [state_Vbattery]
  afbk_A2D_OffsetRod/1 -> [afbk_A2D_OffsetRod]
  ifbk_A2D_OffsetRod/1 -> [ifbk_A2D_OffsetRod]
  calc_Vbattery/1 -> [calc_Vbattery]
  Commands/1(icmd_Base) -> hc_pair_control/1
  hc_pair_control/1 -> hs_OffsetBase/1
  hc_pair_control/2 -> ls_OffsetBase/1
  hc_pair_control/3 -> errorCC_OffsetBase/1
  hc_pair_control/4 -> calc_ifbk_OffsetBase/1
  hc_pair_control/5 -> state_OffsetBase/1
  hc_pair_control1/1 -> hs_OffsetRod/1
  hc_pair_control1/2 -> ls_OffsetRod/1
  hc_pair_control1/3 -> errorCC_OffsetRod/1
  hc_pair_control1/4 -> calc_ifbk_OffsetRod/1
  hc_pair_control1/5 -> state_OffsetRod/1
  Commands/2(icmd_Rod) -> hc_pair_control1/1
  [afbk_A2D_OffsetBase] -> hc_pair_control/3
  [ifbk_A2D_OffsetBase] -> hc_pair_control/4
  [state_Vbattery] -> hc_pair_control/5
  [state_Engine] -> hc_pair_control/6
  [calc_Vbattery] -> hc_pair_control/7
  [afbk_A2D_OffsetRod] -> hc_pair_control1/3
  [ifbk_A2D_OffsetRod] -> hc_pair_control1/4
  [state_Vbattery] -> hc_pair_control1/5
  [state_Engine] -> hc_pair_control1/6
  [calc_Vbattery] -> hc_pair_control1/7
  Compare To Constant/1 -> hc_pair_control1/2, hc_pair_control/2
  ain_PrecRef/1 -> [ain_PrecRef]
  [ain_PrecRef] -> hc_pair_control1/8
  [ain_PrecRef] -> hc_pair_control/8

== system OffsetOutput_harness/VBattery/LP_Filter_Adj_Gain ==
  Gain : Inport
  Input : Inport  Port=2
  LP_Fitler_Adj_Gain : Stateflow chart  TreatAsAtomicUnit=on
  Output : Outport
  wires:
  LP_Fitler_Adj_Gain/1(Output) -> Output/1
  Input/1 -> LP_Fitler_Adj_Gain/2(Input)
  Gain/1 -> LP_Fitler_Adj_Gain/1(Gain)

== system OffsetOutput_harness/VBattery/LP_Filter_Adj_Gain1 ==
  Gain : Inport
  Input : Inport  Port=2
  LP_Fitler_Adj_Gain : Stateflow chart  TreatAsAtomicUnit=on
  Output : Outport
  wires:
  LP_Fitler_Adj_Gain/1(Output) -> Output/1
  Input/1 -> LP_Fitler_Adj_Gain/2(Input)
  Gain/1 -> LP_Fitler_Adj_Gain/1(Gain)

== system OffsetOutput_harness/Feedback/Base Coil/Coil ==
  note: Design Notes:
      |
      | Delta Coil PN??? with  PN??? valve
      |
      | Rfb consists of controller feedback resistor plus harness resistance.
      |
      | Potential Improvements:
      | 1.  Simulate change in coil resistance based on ambient temperature plus
      | temp rise due to current in coil.
      | 2.  Simulate clamping diode which lowers Vin to -0.7Vdc while coil is discharging
  Vin : Inport
  Rcoil : Inport  Port=2
  Divide : Product  Inputs=/*
  Integrator : Integrator
  Lcoil : Constant  Value=.070
  Product : Product  RndMeth=Zero
  Rfb : Constant  Value=.05
  Subtract : Sum
  Sum : Sum  Inputs=|+-
  I : Outport
  wires:
  Rcoil/1 -> Subtract/1
  Rfb/1 -> Subtract/2
  Integrator/1 -> Product/2, I/1  "i"
  Divide/1 -> Integrator/1  "di/dt"
  Lcoil/1 -> Divide/1
  Sum/1 -> Divide/2
  Subtract/1 -> Product/1
  Product/1 -> Sum/2
  Vin/1 -> Sum/1

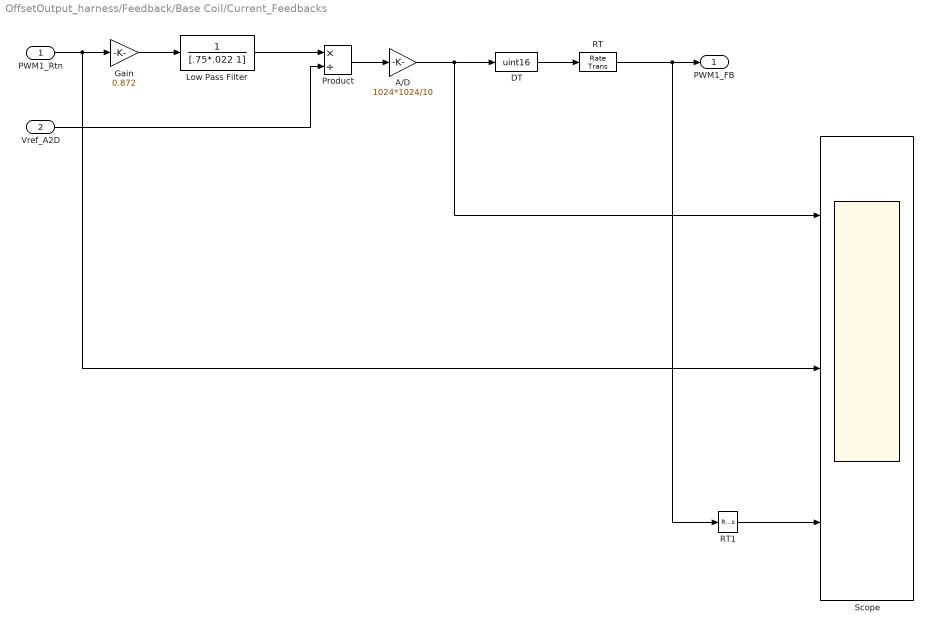
== system OffsetOutput_harness/Feedback/Base Coil/Current_Feedbacks ==
  PWM1_Rtn : Inport
  Vref_A2D : Inport  Port=2
  A/D : Gain  Gain=1024*1024/10
  DT : DataTypeConversion  OutDataTypeStr=uint16
  Gain : Gain  Gain=0.872
  Low Pass Filter : TransferFcn  Denominator=[.75*.022 1]
  Product : Product  Inputs=*/  RndMeth=Zero
  RT : RateTransition  OutPortSampleTime=.01
  RT1 : RateTransition  OutPortSampleTime=0
  Scope : Scope  NumInputPorts=3
      settings: TimeRange=5  YMin=0~-5~-5  YMax=1.4~5~5
  PWM1_FB : Outport
  wires:
  A/D/1 -> Scope/1, DT/1
  Gain/1 -> Low Pass Filter/1
  PWM1_Rtn/1 -> Gain/1, Scope/2
  RT/1 -> PWM1_FB/1, RT1/1
  DT/1 -> RT/1
  Product/1 -> A/D/1
  Low Pass Filter/1 -> Product/1
  RT1/1 -> Scope/3
  Vref_A2D/1 -> Product/2

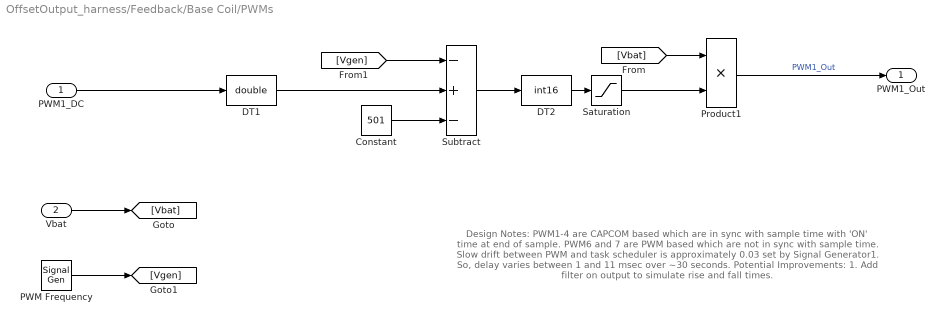
== system OffsetOutput_harness/Feedback/Base Coil/PWMs ==
  note: Design Notes:
      |
      | PWM1-4 are CAPCOM based which are in sync with sample time
      | with 'ON' time at end of sample.
      |
      | PWM6 and 7 are PWM based which are not in sync with sample time.
      | Slow drift between PWM and task scheduler is approximately 0.03
      | set by Signal Generator1.  So, delay varies between 1 and 11 msec
      | over ~30 seconds.
      |
      | Potential Improvements:
      | 1.  Add filter on output to simulate rise and fall times.
  PWM1_DC : Inport
  Vbat : Inport  Port=2  OutDataTypeStr=double
  Constant : Constant  Value=501
  DT1 : DataTypeConversion  OutDataTypeStr=double  SampleTime=0
  DT2 : DataTypeConversion  OutDataTypeStr=int16  SampleTime=0
  PWM Frequency : SignalGenerator  WaveForm=sawtooth  Amplitude=500  Frequency=100
  Product1 : Product  OutDataTypeStr=double  RndMeth=Zero
  Saturation : Saturate  UpperLimit=1  LowerLimit=0
  Subtract : Sum  Inputs=-+-
  PWM1_Out : Outport
  wires:
  Product1/1 -> PWM1_Out/1  "PWM1_Out"
  Subtract/1 -> DT2/1
  DT1/1 -> Subtract/2
  Constant/1 -> Subtract/3
  DT2/1 -> Saturation/1
  Vbat/1 -> [Vbat]
  [Vbat] -> Product1/1
  PWM Frequency/1 -> [Vgen]
  [Vgen] -> Subtract/1
  PWM1_DC/1 -> DT1/1
  Saturation/1 -> Product1/2

== system OffsetOutput_harness/Feedback/Base Coil1/Coil ==
  note: Design Notes:
      |
      | Delta Coil PN??? with  PN??? valve
      |
      | Rfb consists of controller feedback resistor plus harness resistance.
      |
      | Potential Improvements:
      | 1.  Simulate change in coil resistance based on ambient temperature plus
      | temp rise due to current in coil.
      | 2.  Simulate clamping diode which lowers Vin to -0.7Vdc while coil is discharging
  Vin : Inport
  Rcoil : Inport  Port=2
  Divide : Product  Inputs=/*
  Integrator : Integrator
  Lcoil : Constant  Value=.070
  Product : Product  RndMeth=Zero
  Rfb : Constant  Value=.05
  Subtract : Sum
  Sum : Sum  Inputs=|+-
  I : Outport
  wires:
  Rcoil/1 -> Subtract/1
  Rfb/1 -> Subtract/2
  Integrator/1 -> Product/2, I/1  "i"
  Divide/1 -> Integrator/1  "di/dt"
  Lcoil/1 -> Divide/1
  Sum/1 -> Divide/2
  Subtract/1 -> Product/1
  Product/1 -> Sum/2
  Vin/1 -> Sum/1

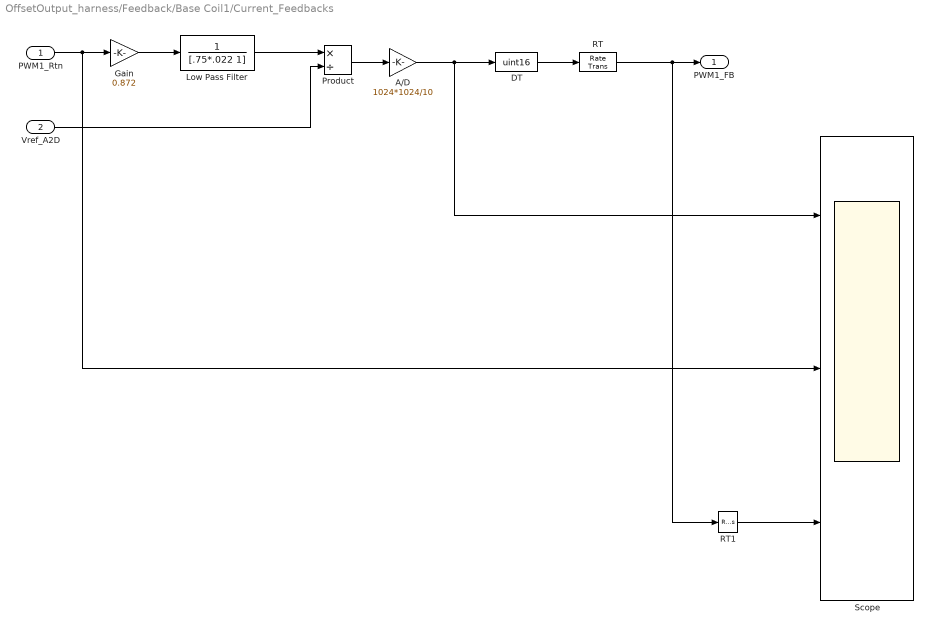
== system OffsetOutput_harness/Feedback/Base Coil1/Current_Feedbacks ==
  PWM1_Rtn : Inport
  Vref_A2D : Inport  Port=2
  A/D : Gain  Gain=1024*1024/10
  DT : DataTypeConversion  OutDataTypeStr=uint16
  Gain : Gain  Gain=0.872
  Low Pass Filter : TransferFcn  Denominator=[.75*.022 1]
  Product : Product  Inputs=*/  RndMeth=Zero
  RT : RateTransition  OutPortSampleTime=.01
  RT1 : RateTransition  OutPortSampleTime=0
  Scope : Scope  NumInputPorts=3
      settings: TimeRange=5  YMin=0~-5~-5  YMax=1.4~5~5
  PWM1_FB : Outport
  wires:
  A/D/1 -> Scope/1, DT/1
  Gain/1 -> Low Pass Filter/1
  PWM1_Rtn/1 -> Gain/1, Scope/2
  RT/1 -> PWM1_FB/1, RT1/1
  DT/1 -> RT/1
  Product/1 -> A/D/1
  Low Pass Filter/1 -> Product/1
  RT1/1 -> Scope/3
  Vref_A2D/1 -> Product/2

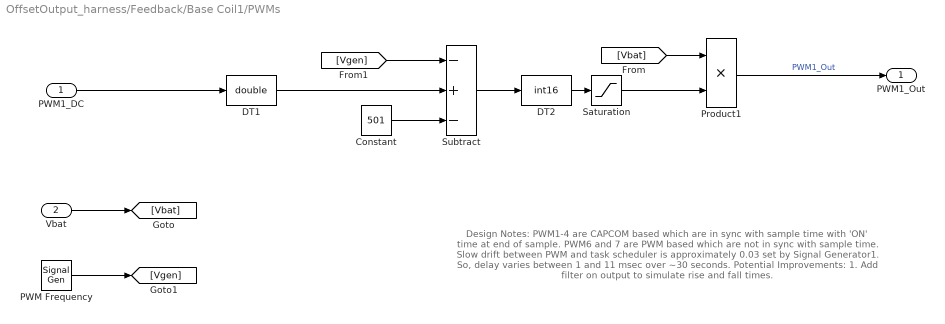
== system OffsetOutput_harness/Feedback/Base Coil1/PWMs ==
  note: Design Notes:
      |
      | PWM1-4 are CAPCOM based which are in sync with sample time
      | with 'ON' time at end of sample.
      |
      | PWM6 and 7 are PWM based which are not in sync with sample time.
      | Slow drift between PWM and task scheduler is approximately 0.03
      | set by Signal Generator1.  So, delay varies between 1 and 11 msec
      | over ~30 seconds.
      |
      | Potential Improvements:
      | 1.  Add filter on output to simulate rise and fall times.
  PWM1_DC : Inport
  Vbat : Inport  Port=2  OutDataTypeStr=double
  Constant : Constant  Value=501
  DT1 : DataTypeConversion  OutDataTypeStr=double  SampleTime=0
  DT2 : DataTypeConversion  OutDataTypeStr=int16  SampleTime=0
  PWM Frequency : SignalGenerator  WaveForm=sawtooth  Amplitude=500  Frequency=100
  Product1 : Product  OutDataTypeStr=double  RndMeth=Zero
  Saturation : Saturate  UpperLimit=1  LowerLimit=0
  Subtract : Sum  Inputs=-+-
  PWM1_Out : Outport
  wires:
  Product1/1 -> PWM1_Out/1  "PWM1_Out"
  Subtract/1 -> DT2/1
  DT1/1 -> Subtract/2
  Constant/1 -> Subtract/3
  DT2/1 -> Saturation/1
  Vbat/1 -> [Vbat]
  [Vbat] -> Product1/1
  PWM Frequency/1 -> [Vgen]
  [Vgen] -> Subtract/1
  PWM1_DC/1 -> DT1/1
  Saturation/1 -> Product1/2

== stateflow chart VBattery/LP_Filter_Adj_Gain/LP_Fitler_Adj_Gain ==
  state INITIAL
    en:Output = Input;
  state LP_FILTER
    du:Output = Output + ((Input - Output)/(1 << Gain));
  (default) -> INITIAL
  INITIAL -> LP_FILTER
  data: Gain input uint8; Input input fixdt(1,16,8); Output output fixdt(1,32,16)

== stateflow chart VBattery/VBattery_State ==
  state NON_FUNCTIONAL
    en:state_VBattery = NORMAL;
    en:state_Alternator = NORMAL;
  state NORMAL
    state NORMAL
      state NORMAL
        en:state_VBattery = NORMAL;
        en:state_Alternator = NORMAL;
      state DEBOUNCE
        en:debounceCount = 0;
        du:debounceCount++;
      (default) -> NORMAL.NORMAL.DEBOUNCE
      NORMAL.NORMAL.DEBOUNCE -> NORMAL.NORMAL.NORMAL : [(debounceCount >= CD_VBATTERY_DEBOUNCE_NORMAL)...
          | || ((state_VBattery == NORMAL) && (state_Alternator == NORMAL))]
    state HIGH
      state HIGH
        en:state_VBattery = HIGH;
        en:state_Alternator = NORMAL;
      state DEBOUNCE
        en:debounceCount = 0;
        du:debounceCount++;
      NORMAL.HIGH.DEBOUNCE -> NORMAL.HIGH.HIGH : [(debounceCount >= CD_VBATTERY_DEBOUNCE_HIGH)...
          | || (state_VBattery == HIGH)]
      (default) -> NORMAL.HIGH.DEBOUNCE
    state EXTREMELY_LOW
      state DEBOUNCE
        en:debounceCount = 0;
        du:debounceCount++;
      state EXTREMELY_LOW
        en:state_VBattery = EXTREMELY_LOW;
        en:state_Alternator = NORMAL;
      NORMAL.EXTREMELY_LOW.DEBOUNCE -> NORMAL.EXTREMELY_LOW.EXTREMELY_LOW : [(debounceCount >= CD_VBATTERY_DEBOUNCE_EXTREMELY_LOW)...
          | || (state_VBattery == EXTREMELY_LOW)]
      (default) -> NORMAL.EXTREMELY_LOW.DEBOUNCE
    state LOW
      state LOW
        en:state_VBattery = LOW;
        en:state_Alternator = NORMAL;
      state DEBOUNCE
        en:debounceCount = 0;
        du:debounceCount++;
      NORMAL.LOW.DEBOUNCE -> NORMAL.LOW.LOW : [(debounceCount >= CD_VBATTERY_DEBOUNCE_LOW)...
          | || (state_VBattery == LOW)]
      (default) -> NORMAL.LOW.DEBOUNCE
    state EXTREMELY_HIGH
      state DEBOUNCE
        en:debounceCount = 0;
        du:debounceCount++;
      state EXTREMELY_HIGH
        en:state_VBattery = EXTREMELY_HIGH;
        en:state_Alternator = NORMAL;
      NORMAL.EXTREMELY_HIGH.DEBOUNCE -> NORMAL.EXTREMELY_HIGH.EXTREMELY_HIGH : [(debounceCount >= CD_VBATTERY_DEBOUNCE_EXTREMELY_HIGH)...
          | || (state_VBattery == EXTREMELY_HIGH)]
      (default) -> NORMAL.EXTREMELY_HIGH.DEBOUNCE
    state ALTERNATOR_LOW
      state DEBOUNCE
        en:debounceCount = 0;
        du:debounceCount++;
      state LOW
        en:state_Alternator = LOW;
        en:state_VBattery = NORMAL;
      (default) -> NORMAL.ALTERNATOR_LOW.DEBOUNCE
      NORMAL.ALTERNATOR_LOW.DEBOUNCE -> NORMAL.ALTERNATOR_LOW.LOW : [(debounceCount >= CD_ALTERNATOR_DEBOUNCE_LOW)]
    state ALTERNATOR_HIGH
      state DEBOUNCE
        en:debounceCount = 0;
        du:debounceCount++;
      state HIGH
        en:state_Alternator = HIGH;
        en:state_VBattery = NORMAL;
      (default) -> NORMAL.ALTERNATOR_HIGH.DEBOUNCE
      NORMAL.ALTERNATOR_HIGH.DEBOUNCE -> NORMAL.ALTERNATOR_HIGH.HIGH : [(debounceCount >= CD_ALTERNATOR_DEBOUNCE_HIGH)]
    NORMAL.EXTREMELY_HIGH -> NORMAL.HIGH [order 2] : [(calc_VBattery < (CD_VBATTERY_EXTREMELY_HIGH - CD_VOLTAGE_HYSTERESIS))...
        | && ((CD_ALTERNATOR_FUNCTION ==NON_FUNCTIONAL)...
        |   || (flt_EngineSpeed < CD_ALTERNATOR_ALARM_ENGINE_SPEED))]
    NORMAL.HIGH -> NORMAL.EXTREMELY_HIGH [order 1] : [(calc_VBattery >= CD_VBATTERY_EXTREMELY_HIGH)]
    (default) -> NORMAL.NORMAL
    NORMAL.HIGH -> NORMAL.NORMAL [order 2] : [(calc_VBattery < (CD_VBATTERY_HIGH - CD_VOLTAGE_HYSTERESIS))]
    NORMAL.NORMAL -> NORMAL.HIGH [order 3] : [(calc_VBattery >= CD_VBATTERY_HIGH)...
        | && ((CD_ALTERNATOR_FUNCTION ==NON_FUNCTIONAL)...
        |    ||  (flt_EngineSpeed < CD_ALTERNATOR_ALARM_ENGINE_SPEED))]
    NORMAL.NORMAL -> NORMAL.LOW [order 4] : [(calc_VBattery <= CD_VBATTERY_LOW)...
        | && ((CD_ALTERNATOR_FUNCTION == NON_FUNCTIONAL)...
        |   ||  (flt_EngineSpeed < CD_ALTERNATOR_ALARM_ENGINE_SPEED))]
    NORMAL.LOW -> NORMAL.NORMAL [order 1] : [(calc_VBattery > (CD_VBATTERY_LOW + CD_VOLTAGE_HYSTERESIS))...
        | && (state_Engine != ENGINE_CRANKING)]
    NORMAL.LOW -> NORMAL.EXTREMELY_LOW [order 2] : [(calc_VBattery <= CD_VBATTERY_EXTREMELY_LOW)]
    NORMAL.EXTREMELY_LOW -> NORMAL.LOW [order 2] : [(calc_VBattery > (CD_VBATTERY_EXTREMELY_LOW + CD_VOLTAGE_HYSTERESIS))...
        | && (state_Engine != ENGINE_CRANKING)...
        | && ((CD_ALTERNATOR_FUNCTION == NON_FUNCTIONAL)...
        |   ||  (flt_EngineSpeed < CD_ALTERNATOR_ALARM_ENGINE_SPEED))]
    NORMAL.NORMAL -> ALTERNATOR_LOW [order 1] : [(CD_ALTERNATOR_FUNCTION != NON_FUNCTIONAL)...
        | && (calc_VBattery <= CD_ALTERNATOR_LOW)...
        | && (flt_EngineSpeed >= CD_ALTERNATOR_ALARM_ENGINE_SPEED)]
    ALTERNATOR_LOW -> NORMAL.NORMAL [order 1] : [(calc_VBattery > (CD_ALTERNATOR_LOW + CD_VOLTAGE_HYSTERESIS))...
        | || (flt_EngineSpeed < CD_ALTERNATOR_ALARM_ENGINE_SPEED)]
    NORMAL.NORMAL -> ALTERNATOR_HIGH [order 2] : [(CD_ALTERNATOR_FUNCTION != NON_FUNCTIONAL)...
        | && (calc_VBattery >= CD_ALTERNATOR_HIGH)...
        | && (flt_EngineSpeed >= CD_ALTERNATOR_ALARM_ENGINE_SPEED)]
    ALTERNATOR_HIGH -> NORMAL.NORMAL [order 1] : [(calc_VBattery < (CD_ALTERNATOR_HIGH - CD_VOLTAGE_HYSTERESIS))...
        | || (flt_EngineSpeed < CD_ALTERNATOR_ALARM_ENGINE_SPEED)]
    NORMAL.EXTREMELY_LOW -> ALTERNATOR_LOW [order 1] : [(calc_VBattery > (CD_VBATTERY_EXTREMELY_LOW + CD_VOLTAGE_HYSTERESIS))...
        | && ((CD_ALTERNATOR_FUNCTION != NON_FUNCTIONAL) && (flt_EngineSpeed >= CD_ALTERNATOR_ALARM_ENGINE_SPEED))]
    ALTERNATOR_LOW -> NORMAL.EXTREMELY_LOW [order 2] : [(calc_VBattery <= CD_VBATTERY_EXTREMELY_LOW)]
    ALTERNATOR_HIGH -> NORMAL.EXTREMELY_HIGH [order 2] : [(calc_VBattery >= CD_VBATTERY_EXTREMELY_HIGH)]
    NORMAL.EXTREMELY_HIGH -> ALTERNATOR_HIGH [order 1] : [(calc_VBattery < (CD_VBATTERY_EXTREMELY_HIGH - CD_VOLTAGE_HYSTERESIS))...
        | && ((CD_ALTERNATOR_FUNCTION != NON_FUNCTIONAL) && (flt_EngineSpeed >= CD_ALTERNATOR_ALARM_ENGINE_SPEED))]
  state OORL
    state DEBOUNCE_OORL
      en:debounceCount = 0;
      du:debounceCount++;
    state OORL
      en:state_VBattery = OORL;
      en:state_Alternator = NORMAL;
    DEBOUNCE_OORL -> OORL.OORL : [(debounceCount >= CD_VBATTERY_DEBOUNCE_OORL)...
        | || (state_VBattery == OORL)]
    (default) -> DEBOUNCE_OORL
  (default) -> NON_FUNCTIONAL
  NORMAL -> OORL : [(calc_VBattery <= CD_VBATTERY_OORL)]
  OORL -> NORMAL : [(state_Engine != ENGINE_CRANKING)...
      | && (calc_VBattery > (CD_VBATTERY_OORL + CD_VOLTAGE_HYSTERESIS))]
  NON_FUNCTIONAL -> NORMAL : [(CD_VBATTERY_FUNCTION != NON_FUNCTIONAL)]
  data: state_VBattery output uint8; calc_VBattery input fixdt(0,16,8); debounceCount local uint16 =0; CD_VBATTERY_DEBOUNCE_EXTREMELY_LOW parameter uint16; CD_VBATTERY_DEBOUNCE_HIGH parameter uint16; CD_VBATTERY_DEBOUNCE_LOW parameter uint16; CD_VBATTERY_DEBOUNCE_NORMAL parameter uint16; CD_VBATTERY_DEBOUNCE_OORL parameter uint16; CD_VBATTERY_EXTREMELY_LOW parameter uint16; CD_VBATTERY_FUNCTION parameter uint8; CD_VBATTERY_HIGH parameter uint8; CD_VBATTERY_LOW parameter uint8; CD_VBATTERY_OORL parameter uint8; state_Engine input uint8; CD_VBATTERY_EXTREMELY_HIGH parameter uint8; CD_VBATTERY_DEBOUNCE_EXTREMELY_HIGH parameter uint16; HIGH parameter uint8 =10; OORL parameter uint8 =22; LOW parameter uint8 =9; NORMAL parameter uint8 =8; EXTREMELY_LOW parameter uint8 =14; EXTREMELY_HIGH parameter uint8 =11; ENGINE_CRANKING parameter uint8 =2; NON_FUNCTIONAL parameter uint8 =255; CD_VOLTAGE_HYSTERESIS parameter fixdt(0,8,4); CD_ALTERNATOR_FUNCTION parameter uint8; CD_ALTERNATOR_HIGH parameter uint8; CD_ALTERNATOR_LOW parameter uint8; state_Alternator output uint8; CD_ALTERNATOR_ALARM_ENGINE_SPEED parameter uint16; flt_EngineSpeed input uint16; CD_ALTERNATOR_DEBOUNCE_HIGH parameter uint16; CD_ALTERNATOR_DEBOUNCE_LOW parameter uint16

== stateflow chart Offset/Offset/Commands ==
  state Active
    state Neutral
      en:
      icmd_Base = 0;
      icmd_Rod = 0;
    state RodActive
      en:
      icmd_Base = 0;
      icmd_Rod = icmd_In;
      du:
      icmd_Rod = icmd_In;
    state BaseActive
      en:
      icmd_Rod = 0;
      icmd_Base = icmd_In;
      du:
      icmd_Base = icmd_In;
    Neutral -> BaseActive [order 2] : [state_OffsetPot == BASE_ACTIVE]
    (default) -> Neutral
    Neutral -> RodActive [order 1] : [state_OffsetPot == ROD_ACTIVE]
    RodActive -> Neutral [order 1] : [state_OffsetPot != BASE_ACTIVE &&...
        |  state_OffsetPot != ROD_ACTIVE]
    BaseActive -> RodActive [order 2] : [state_OffsetPot == ROD_ACTIVE]
    RodActive -> BaseActive [order 2] : [state_OffsetPot == BASE_ACTIVE]
    BaseActive -> Neutral [order 1] : [state_OffsetPot != BASE_ACTIVE &&...
        |  state_OffsetPot != ROD_ACTIVE]
  state Inactive
    en:
    icmd_Base = 0;
    icmd_Rod = 0;
  Active -> Inactive : [state_Console != ACTIVE ||...
      |  state_Engine == ENGINE_CRANKING]
  Inactive -> Active : [state_Console == ACTIVE &&...
      |  state_Engine != ENGINE_CRANKING]
  (default) -> Inactive
  data: icmd_In input fixdt(0,16,12); state_OffsetPot input uint8; state_Engine input uint8; ENGINE_CRANKING parameter uint8; icmd_Base output fixdt(0,16,12); BASE_ACTIVE parameter uint8; ROD_ACTIVE parameter uint8; ACTIVE parameter uint8; state_Console input uint8; icmd_Rod output fixdt(0,16,12)

== stateflow chart VBattery/LP_Filter_Adj_Gain1/LP_Fitler_Adj_Gain ==
  state INITIAL
    en:Output = Input;
  state LP_FILTER
    du:Output = Output + ((Input - Output)/(1 << Gain));
  (default) -> INITIAL
  INITIAL -> LP_FILTER
  data: Gain input uint8; Input input fixdt(1,16,8); Output output fixdt(1,32,16)
